simulink model "gm_soc_dvbs2_fpga"  (R2025b)
settings: Solver=VariableStepAuto  StartTime=0.0  StopTime=10.0  RelTol=1e-3
InitFcn:
  | soc_dvbs2_init;
undefined symbols (not defined in the file or in its folder): Add, coefficientsLog, coefficientsSqrt1, coefficientsSqrt2, dataBits, Deinterleaver, designMultirateFIR, noisePow, Shift, Short, soc_dvbs2_designFIRFilter, soc_dvbs2_txPacketBits, syncWord, txDataOut, txFiltCoeff, XData
libraries: simulink x304, hdlsllib x265, dspsigops x15, dsphdlfiltering2 x8, hdlmdlgenlib x6, dsphdlsigops2 x5, commseqgen3 x5, dsphdlmathfun2 x3, hwlogicconnlib x2, whdledac x2, commhdlcrc x2, whdlutilities x1
(part 16 of 36)

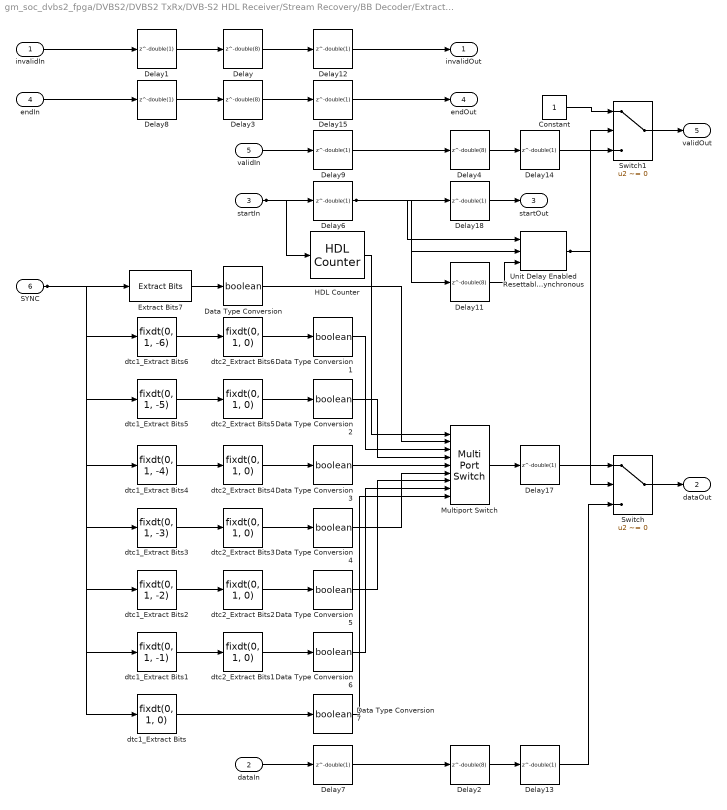
== system gm_soc_dvbs2_fpga/DVBS2/DVBS2 TxRx/DVB-S2 HDL Receiver/Stream Recovery/BB Decoder/Extract Stream/Insert SYNC ==
  invalidIn : Inport  OutDataTypeStr=boolean  PortDimensions=1  SampleTime=7.8125e-09
  dataIn : Inport  Port=2  OutDataTypeStr=boolean  PortDimensions=1  SampleTime=7.8125e-09
  startIn : Inport  Port=3  OutDataTypeStr=boolean  PortDimensions=1  SampleTime=7.8125e-09
  endIn : Inport  Port=4  OutDataTypeStr=boolean  PortDimensions=1  SampleTime=7.8125e-09
  validIn : Inport  Port=5  OutDataTypeStr=boolean  PortDimensions=1  SampleTime=7.8125e-09
  SYNC : Inport  Port=6  OutDataTypeStr=uint8  PortDimensions=1  SampleTime=7.8125e-09
  Constant : Constant  OutDataTypeStr=boolean  SampleTime=7.8125e-09
  Data Type Conversion{,1..7} (8 alike) : DataTypeConversion  OutDataTypeStr=boolean  SampleTime=7.8125e-09  SaturateOnIntegerOverflow=off  RndMeth=Floor
  Delay{,2..4,11} (5 alike) : Delay  DelayLength=double(8)  InitialCondition=0  SampleTime=7.8125e-09
  Delay{1,6..9,12..15,17..18} (11 alike) : Delay  DelayLength=double(1)  InitialCondition=0  SampleTime=7.8125e-09
  Extract Bits7 : simulink/Logic and Bit Operations/Extract Bits  bitsToExtract=Range of bits  numBits=8  bitIdxRange=[7 7]  outScalingMode=Treat bit field as an integer
  HDL Counter : hdlsllib/Sources/HDL Counter  CountType=Count limited  CountInit=0  CountStep=1  CountMax=7  CountFromType=Initial value  CountFrom=0  CountResetPort=on  CountLoadPort=off  CountEnbPort=off  CountDirPort=off  CountHitOutputPort=off  CountDataType=Unsigned  CountWordLen=3  CountFracLen=0  CountSampTime=1
  Multiport Switch : MultiPortSwitch  DataPortOrder=Zero-based contiguous  Inputs=8  DiagnosticForDefault=None  zeroidx=on  SampleTime=7.8125e-09  SaturateOnIntegerOverflow=off  InputSameDT=off
  Switch : Switch  Criteria=u2 ~= 0  Threshold="fi(0,0,1,0,\"hex\",\"0\")"  OutDataTypeStr=boolean  SampleTime=7.8125e-09  SaturateOnIntegerOverflow=off  InputSameDT=off
  Switch1 : Switch  Criteria=u2 ~= 0  Threshold="fi(0,0,1,0,\"hex\",\"0\")"  OutDataTypeStr=boolean  SampleTime=7.8125e-09  SaturateOnIntegerOverflow=off  InputSameDT=off
  Unit Delay Enabled Resettable Synchronous : hdlsllib/Discrete/Unit Delay Enabled Resettable Synchronous  InitialCondition=double(0)  SampleTime=-1
  dtc1_Extract Bits : DataTypeConversion  OutDataTypeStr=fixdt(0, 1, 0)  SampleTime=7.8125e-09  SaturateOnIntegerOverflow=off  RndMeth=Floor
  dtc1_Extract Bits1 : DataTypeConversion  OutDataTypeStr=fixdt(0, 1, -1)  SampleTime=7.8125e-09  SaturateOnIntegerOverflow=off  RndMeth=Floor
  dtc1_Extract Bits2 : DataTypeConversion  OutDataTypeStr=fixdt(0, 1, -2)  SampleTime=7.8125e-09  SaturateOnIntegerOverflow=off  RndMeth=Floor
  dtc1_Extract Bits3 : DataTypeConversion  OutDataTypeStr=fixdt(0, 1, -3)  SampleTime=7.8125e-09  SaturateOnIntegerOverflow=off  RndMeth=Floor
  dtc1_Extract Bits4 : DataTypeConversion  OutDataTypeStr=fixdt(0, 1, -4)  SampleTime=7.8125e-09  SaturateOnIntegerOverflow=off  RndMeth=Floor
  dtc1_Extract Bits5 : DataTypeConversion  OutDataTypeStr=fixdt(0, 1, -5)  SampleTime=7.8125e-09  SaturateOnIntegerOverflow=off  RndMeth=Floor
  dtc1_Extract Bits6 : DataTypeConversion  OutDataTypeStr=fixdt(0, 1, -6)  SampleTime=7.8125e-09  SaturateOnIntegerOverflow=off  RndMeth=Floor
  dtc2_Extract Bits{1..6} (6 alike) : DataTypeConversion  OutDataTypeStr=fixdt(0, 1, 0)  ConvertRealWorld=Stored Integer (SI)  SampleTime=7.8125e-09  SaturateOnIntegerOverflow=off  RndMeth=Floor
  invalidOut : Outport  SampleTime=7.8125e-09
  dataOut : Outport  Port=2  SampleTime=7.8125e-09
  startOut : Outport  Port=3  SampleTime=7.8125e-09
  endOut : Outport  Port=4  SampleTime=7.8125e-09
  validOut : Outport  Port=5  SampleTime=7.8125e-09
  wires:
  dtc1_Extract Bits5/1 -> dtc2_Extract Bits5/1
  Data Type Conversion3/1 -> Multiport Switch/5
  Delay/1 -> Delay12/1
  dtc1_Extract Bits6/1 -> dtc2_Extract Bits6/1
  Data Type Conversion7/1 -> Multiport Switch/9
  invalidIn/1 -> Delay1/1
  dtc2_Extract Bits2/1 -> Data Type Conversion5/1
  SYNC/1 -> dtc1_Extract Bits6/1, dtc1_Extract Bits4/1, Extract Bits7/1, dtc1_Extract Bits3/1, dtc1_Extract Bits2/1, dtc1_Extract Bits1/1, dtc1_Extract Bits5/1, dtc1_Extract Bits/1
  Data Type Conversion6/1 -> Multiport Switch/8
  endIn/1 -> Delay8/1
  Delay12/1 -> invalidOut/1
  Delay1/1 -> Delay/1
  Delay8/1 -> Delay3/1
  Extract Bits7/1 -> Data Type Conversion/1
  dtc1_Extract Bits4/1 -> dtc2_Extract Bits4/1
  dtc1_Extract Bits3/1 -> dtc2_Extract Bits3/1
  validIn/1 -> Delay9/1
  dtc1_Extract Bits2/1 -> dtc2_Extract Bits2/1
  dtc1_Extract Bits1/1 -> dtc2_Extract Bits1/1
  dtc1_Extract Bits/1 -> Data Type Conversion7/1
  Delay3/1 -> Delay15/1
  Data Type Conversion5/1 -> Multiport Switch/7
  startIn/1 -> Delay6/1, HDL Counter/1
  Data Type Conversion/1 -> Multiport Switch/2
  Data Type Conversion4/1 -> Multiport Switch/6
  dtc2_Extract Bits6/1 -> Data Type Conversion1/1
  Data Type Conversion2/1 -> Multiport Switch/4
  dtc2_Extract Bits5/1 -> Data Type Conversion2/1
  dataIn/1 -> Delay7/1
  dtc2_Extract Bits4/1 -> Data Type Conversion3/1
  Constant/1 -> Switch1/1
  dtc2_Extract Bits3/1 -> Data Type Conversion4/1
  dtc2_Extract Bits1/1 -> Data Type Conversion6/1
  Delay15/1 -> endOut/1
  Delay9/1 -> Delay4/1
  Delay6/1 -> Unit Delay Enabled Resettable Synchronous/1, Unit Delay Enabled Resettable Synchronous/2, Delay18/1, Delay11/1
  HDL Counter/1 -> Multiport Switch/1
  Data Type Conversion1/1 -> Multiport Switch/3
  Delay7/1 -> Delay2/1
  Unit Delay Enabled Resettable Synchronous/1 -> Switch1/2, Switch/2
  Delay4/1 -> Delay14/1
  Delay18/1 -> startOut/1
  Switch1/1 -> validOut/1
  Delay11/1 -> Unit Delay Enabled Resettable Synchronous/3
  Multiport Switch/1 -> Delay17/1
  Delay2/1 -> Delay13/1
  Delay14/1 -> Switch1/3
  Delay17/1 -> Switch/1
  Delay13/1 -> Switch/3
  Switch/1 -> dataOut/1

== system gm_soc_dvbs2_fpga/DVBS2/DVBS2 TxRx/DVB-S2 HDL Receiver/Synchronizer and PL Header Decoder/Fine Phase Synchronizer/Power Q and Beta Offset Rotation/Complex Multiplier ==
  In1 : Inport  OutDataTypeStr=fixdt(1, 22, 14)  PortDimensions=1  SampleTime=2.5e-07
      settings: SignalType=complex
  In2 : Inport  Port=2  OutDataTypeStr=fixdt(1, 22, 14)  PortDimensions=1  SampleTime=2.5e-07
      settings: SignalType=complex
  AddADn : Sum  Inputs=++|  OutDataTypeStr=fixdt(1, 22, 14)
  AddAUp : Sum  Inputs=|+-  OutDataTypeStr=fixdt(1, 22, 14)
  AddBCtr : Sum  Inputs=+|+  OutDataTypeStr=fixdt(1, 23, 14)
  AddBDn : Sum  Inputs=|+-  OutDataTypeStr=fixdt(1, 23, 14)
  AddBUp : Sum  Inputs=++|  OutDataTypeStr=fixdt(1, 23, 14)
  Complex to Real-Imag : ComplexToRealImag
  Complex to Real-Imag1 : ComplexToRealImag
  Delay{1..8,21} (9 alike) : Delay
  Delay{9..20} (12 alike) : Delay  DelayLength=1
  ProductCtr : Product  OutDataTypeStr=fixdt(1, 45, 28)
  ProductDn : Product  OutDataTypeStr=fixdt(1, 45, 28)
  ProductUp : Product  OutDataTypeStr=fixdt(1, 45, 28)
  Real-Imag to Complex : RealImagToComplex
  Out1 : Outport  SampleTime=2.5e-07  VectorParamsAs1DForOutWhenUnconnected=off
  wires:
  Delay9/1 -> AddBUp/1
  Delay7/1 -> Delay17/1
  ProductUp/1 -> Delay21/1
  AddBDn/1 -> Delay5/1
  [IM2] -> Delay15/1
  [RE2] -> Delay14/1
  Delay5/1 -> ProductDn/2
  [IM2] -> Delay10/1
  AddAUp/1 -> Delay19/1
  ProductCtr/1 -> Delay7/1
  Complex to Real-Imag/2 -> Delay13/1
  [RE2] -> Delay9/1
  Delay11/1 -> AddBCtr/1, Delay1/1
  In1/1 -> Complex to Real-Imag/1
  Delay10/1 -> AddBUp/2
  Delay12/1 -> Delay3/1
  In2/1 -> Complex to Real-Imag1/1
  Complex to Real-Imag/1 -> Delay11/1
  Complex to Real-Imag1/1 -> [RE2]
  Complex to Real-Imag1/2 -> [IM2]
  Delay14/1 -> AddBDn/1
  Delay15/1 -> AddBDn/2
  AddADn/1 -> Delay20/1
  AddBUp/1 -> Delay8/1
  ProductDn/1 -> Delay6/1
  AddBCtr/1 -> Delay2/1
  [IM2] -> Delay12/1
  Delay13/1 -> AddBCtr/2, Delay4/1
  Delay8/1 -> ProductUp/1
  Delay1/1 -> ProductUp/2
  Delay4/1 -> ProductDn/1
  Delay2/1 -> ProductCtr/1
  Delay3/1 -> ProductCtr/2
  Delay21/1 -> Delay16/1
  Delay6/1 -> Delay18/1
  Delay18/1 -> AddADn/2
  Delay16/1 -> AddAUp/1
  Delay17/1 -> AddAUp/2, AddADn/1
  Delay19/1 -> Real-Imag to Complex/1
  Delay20/1 -> Real-Imag to Complex/2
  Real-Imag to Complex/1 -> Out1/1

== system gm_soc_dvbs2_fpga/DVBS2/DVBS2 TxRx/DVB-S2 HDL Receiver/Synchronizer and PL Header Decoder/Fine Phase Synchronizer/Power Q and Beta Offset Rotation/Complex Multiplier1 ==
  In1 : Inport  OutDataTypeStr=fixdt(1, 22, 14)  PortDimensions=1  SampleTime=2.5e-07
      settings: SignalType=complex
  In2 : Inport  Port=2  OutDataTypeStr=fixdt(1, 22, 14)  PortDimensions=1  SampleTime=2.5e-07
      settings: SignalType=complex
  AddADn : Sum  Inputs=++|  OutDataTypeStr=fixdt(1, 22, 14)
  AddAUp : Sum  Inputs=|+-  OutDataTypeStr=fixdt(1, 22, 14)
  AddBCtr : Sum  Inputs=+|+  OutDataTypeStr=fixdt(1, 23, 14)
  AddBDn : Sum  Inputs=|+-  OutDataTypeStr=fixdt(1, 23, 14)
  AddBUp : Sum  Inputs=++|  OutDataTypeStr=fixdt(1, 23, 14)
  Complex to Real-Imag : ComplexToRealImag
  Complex to Real-Imag1 : ComplexToRealImag
  Delay{1..8,21} (9 alike) : Delay
  Delay{9..20} (12 alike) : Delay  DelayLength=1
  ProductCtr : Product  OutDataTypeStr=fixdt(1, 45, 28)
  ProductDn : Product  OutDataTypeStr=fixdt(1, 45, 28)
  ProductUp : Product  OutDataTypeStr=fixdt(1, 45, 28)
  Real-Imag to Complex : RealImagToComplex
  Out1 : Outport  SampleTime=2.5e-07  VectorParamsAs1DForOutWhenUnconnected=off
  wires:
  Real-Imag to Complex/1 -> Out1/1
  ProductUp/1 -> Delay21/1
  AddBDn/1 -> Delay5/1
  [IM2] -> Delay15/1
  [RE2] -> Delay14/1
  [IM2] -> Delay10/1
  AddAUp/1 -> Delay19/1
  ProductCtr/1 -> Delay7/1
  Complex to Real-Imag/2 -> Delay13/1
  [RE2] -> Delay9/1
  In1/1 -> Complex to Real-Imag/1
  Delay10/1 -> AddBUp/2
  Delay12/1 -> Delay3/1
  In2/1 -> Complex to Real-Imag1/1
  Delay20/1 -> Real-Imag to Complex/2
  Delay9/1 -> AddBUp/1
  Complex to Real-Imag/1 -> Delay11/1
  Complex to Real-Imag1/1 -> [RE2]
  ProductDn/1 -> Delay6/1
  AddBCtr/1 -> Delay2/1
  [IM2] -> Delay12/1
  Complex to Real-Imag1/2 -> [IM2]
  Delay14/1 -> AddBDn/1
  Delay15/1 -> AddBDn/2
  AddADn/1 -> Delay20/1
  AddBUp/1 -> Delay8/1
  Delay19/1 -> Real-Imag to Complex/1
  Delay11/1 -> AddBCtr/1, Delay1/1
  Delay13/1 -> AddBCtr/2, Delay4/1
  Delay8/1 -> ProductUp/1
  Delay1/1 -> ProductUp/2
  Delay4/1 -> ProductDn/1
  Delay5/1 -> ProductDn/2
  Delay2/1 -> ProductCtr/1
  Delay3/1 -> ProductCtr/2
  Delay21/1 -> Delay16/1
  Delay6/1 -> Delay18/1
  Delay16/1 -> AddAUp/1
  Delay7/1 -> Delay17/1
  Delay17/1 -> AddAUp/2, AddADn/1
  Delay18/1 -> AddADn/2

== system gm_soc_dvbs2_fpga/DVBS2/DVBS2 TxRx/DVB-S2 HDL Receiver/Synchronizer and PL Header Decoder/Fine Phase Synchronizer/Power Q and Beta Offset Rotation/Complex Multiplier2 ==
  In1 : Inport  OutDataTypeStr=fixdt(1, 22, 14)  PortDimensions=1  SampleTime=2.5e-07
      settings: SignalType=complex
  In2 : Inport  Port=2  OutDataTypeStr=fixdt(1, 22, 14)  PortDimensions=1  SampleTime=2.5e-07
      settings: SignalType=complex
  AddADn : Sum  Inputs=++|  OutDataTypeStr=fixdt(1, 22, 14)
  AddAUp : Sum  Inputs=|+-  OutDataTypeStr=fixdt(1, 22, 14)
  AddBCtr : Sum  Inputs=+|+  OutDataTypeStr=fixdt(1, 23, 14)
  AddBDn : Sum  Inputs=|+-  OutDataTypeStr=fixdt(1, 23, 14)
  AddBUp : Sum  Inputs=++|  OutDataTypeStr=fixdt(1, 23, 14)
  Complex to Real-Imag : ComplexToRealImag
  Complex to Real-Imag1 : ComplexToRealImag
  Delay{1..8,21} (9 alike) : Delay
  Delay{9..20} (12 alike) : Delay  DelayLength=1
  ProductCtr : Product  OutDataTypeStr=fixdt(1, 45, 28)
  ProductDn : Product  OutDataTypeStr=fixdt(1, 45, 28)
  ProductUp : Product  OutDataTypeStr=fixdt(1, 45, 28)
  Real-Imag to Complex : RealImagToComplex
  Out1 : Outport  SampleTime=2.5e-07  VectorParamsAs1DForOutWhenUnconnected=off
  wires:
  Delay20/1 -> Real-Imag to Complex/2
  Delay9/1 -> AddBUp/1
  Delay7/1 -> Delay17/1
  [IM2] -> Delay15/1
  [RE2] -> Delay14/1
  Delay5/1 -> ProductDn/2
  [IM2] -> Delay10/1
  [RE2] -> Delay9/1
  In1/1 -> Complex to Real-Imag/1
  In2/1 -> Complex to Real-Imag1/1
  Delay10/1 -> AddBUp/2
  Complex to Real-Imag/1 -> Delay11/1
  AddAUp/1 -> Delay19/1
  ProductCtr/1 -> Delay7/1
  Complex to Real-Imag/2 -> Delay13/1
  Complex to Real-Imag1/1 -> [RE2]
  ProductDn/1 -> Delay6/1
  AddBCtr/1 -> Delay2/1
  Complex to Real-Imag1/2 -> [IM2]
  Delay14/1 -> AddBDn/1
  Delay15/1 -> AddBDn/2
  AddADn/1 -> Delay20/1
  AddBUp/1 -> Delay8/1
  Delay19/1 -> Real-Imag to Complex/1
  Delay11/1 -> AddBCtr/1, Delay1/1
  [IM2] -> Delay12/1
  Delay13/1 -> AddBCtr/2, Delay4/1
  Real-Imag to Complex/1 -> Out1/1
  ProductUp/1 -> Delay21/1
  AddBDn/1 -> Delay5/1
  Delay8/1 -> ProductUp/1
  Delay1/1 -> ProductUp/2
  Delay12/1 -> Delay3/1
  Delay4/1 -> ProductDn/1
  Delay2/1 -> ProductCtr/1
  Delay3/1 -> ProductCtr/2
  Delay21/1 -> Delay16/1
  Delay6/1 -> Delay18/1
  Delay18/1 -> AddADn/2
  Delay16/1 -> AddAUp/1
  Delay17/1 -> AddAUp/2, AddADn/1

== system gm_soc_dvbs2_fpga/DVBS2/DVBS2 TxRx/DVB-S2 HDL Receiver/Synchronizer and PL Header Decoder/Fine Phase Synchronizer/Power Q and Beta Offset Rotation/Gain ==
  In1 : Inport  OutDataTypeStr=fixdt(1, 22, 14)  PortDimensions=1  SampleTime=2.5e-07
      settings: SignalType=complex
  AddADn : Sum  Inputs=++|  OutDataTypeStr=fixdt(1, 22, 14)
  AddAUp : Sum  Inputs=|+-  OutDataTypeStr=fixdt(1, 22, 14)
  AddBCtr : Sum  Inputs=+|+  OutDataTypeStr=fixdt(1, 23, 14)
  AddBDn : Sum  Inputs=|+-  OutDataTypeStr=fixdt(1, 17, 15)
  AddBUp : Sum  Inputs=++|  OutDataTypeStr=fixdt(1, 17, 15)
  Complex to Real-Imag : ComplexToRealImag
  Complex to Real-Imag1 : ComplexToRealImag
  Constant : Constant  Value=fi(exp(1i*pi/4),1,16)  OutDataTypeStr=fixdt(1, 16, 15)  SampleTime=-1
  Delay{1..8,21} (9 alike) : Delay
  Delay{9..20} (12 alike) : Delay  DelayLength=1
  ProductCtr : Product  OutDataTypeStr=fixdt(1, 39, 29)
  ProductDn : Product  OutDataTypeStr=fixdt(1, 39, 29)
  ProductUp : Product  OutDataTypeStr=fixdt(1, 39, 29)
  Real-Imag to Complex : RealImagToComplex
  Out1 : Outport  SampleTime=2.5e-07  VectorParamsAs1DForOutWhenUnconnected=off
  wires:
  Delay9/1 -> AddBUp/1
  Delay7/1 -> Delay17/1
  ProductUp/1 -> Delay21/1
  [IM2] -> Delay15/1
  Delay20/1 -> Real-Imag to Complex/2
  [RE2] -> Delay14/1
  Delay5/1 -> ProductDn/2
  [IM2] -> Delay10/1
  ProductCtr/1 -> Delay7/1
  [RE2] -> Delay9/1
  Delay10/1 -> AddBUp/2
  Constant/1 -> Complex to Real-Imag1/1
  In1/1 -> Complex to Real-Imag/1
  Complex to Real-Imag/1 -> Delay11/1
  AddAUp/1 -> Delay19/1
  Complex to Real-Imag/2 -> Delay13/1
  Complex to Real-Imag1/1 -> [RE2]
  AddBCtr/1 -> Delay2/1
  Complex to Real-Imag1/2 -> [IM2]
  Delay14/1 -> AddBDn/1
  Delay15/1 -> AddBDn/2
  AddBUp/1 -> Delay8/1
  Delay11/1 -> Delay1/1, AddBCtr/1
  ProductDn/1 -> Delay6/1
  [IM2] -> Delay12/1
  Delay13/1 -> AddBCtr/2, Delay4/1
  Real-Imag to Complex/1 -> Out1/1
  AddBDn/1 -> Delay5/1
  Delay8/1 -> ProductUp/1
  Delay1/1 -> ProductUp/2
  Delay12/1 -> Delay3/1
  Delay4/1 -> ProductDn/1
  Delay2/1 -> ProductCtr/1
  AddADn/1 -> Delay20/1
  Delay3/1 -> ProductCtr/2
  Delay21/1 -> Delay16/1
  Delay6/1 -> Delay18/1
  Delay16/1 -> AddAUp/1
  Delay17/1 -> AddADn/1, AddAUp/2
  Delay18/1 -> AddADn/2
  Delay19/1 -> Real-Imag to Complex/1

== system gm_soc_dvbs2_fpga/DVBS2/DVBS2 TxRx/DVB-S2 HDL Receiver/Synchronizer and PL Header Decoder/Fine Phase Synchronizer/Power Q and Beta Offset Rotation/Gain1 ==
  In1 : Inport  OutDataTypeStr=fixdt(1, 22, 14)  PortDimensions=1  SampleTime=2.5e-07
      settings: SignalType=complex
  AddADn : Sum  Inputs=++|  OutDataTypeStr=fixdt(1, 22, 14)
  AddAUp : Sum  Inputs=|+-  OutDataTypeStr=fixdt(1, 22, 14)
  AddBCtr : Sum  Inputs=+|+  OutDataTypeStr=fixdt(1, 23, 14)
  AddBDn : Sum  Inputs=|+-  OutDataTypeStr=fixdt(1, 17, 15)
  AddBUp : Sum  Inputs=++|  OutDataTypeStr=fixdt(1, 17, 15)
  Complex to Real-Imag : ComplexToRealImag
  Complex to Real-Imag1 : ComplexToRealImag
  Constant : Constant  Value=fi(exp(1i*pi/4),1,16)  OutDataTypeStr=fixdt(1, 16, 15)  SampleTime=-1
  Delay{1..8,21} (9 alike) : Delay
  Delay{9..20} (12 alike) : Delay  DelayLength=1
  ProductCtr : Product  OutDataTypeStr=fixdt(1, 39, 29)
  ProductDn : Product  OutDataTypeStr=fixdt(1, 39, 29)
  ProductUp : Product  OutDataTypeStr=fixdt(1, 39, 29)
  Real-Imag to Complex : RealImagToComplex
  Out1 : Outport  SampleTime=2.5e-07  VectorParamsAs1DForOutWhenUnconnected=off
  wires:
  Delay9/1 -> AddBUp/1
  Delay7/1 -> Delay17/1
  ProductUp/1 -> Delay21/1
  AddBDn/1 -> Delay5/1
  [IM2] -> Delay15/1
  [RE2] -> Delay14/1
  Delay5/1 -> ProductDn/2
  [IM2] -> Delay10/1
  AddAUp/1 -> Delay19/1
  ProductCtr/1 -> Delay7/1
  [RE2] -> Delay9/1
  Delay10/1 -> AddBUp/2
  Constant/1 -> Complex to Real-Imag1/1
  In1/1 -> Complex to Real-Imag/1
  Complex to Real-Imag/1 -> Delay11/1
  Complex to Real-Imag/2 -> Delay13/1
  Complex to Real-Imag1/1 -> [RE2]
  Complex to Real-Imag1/2 -> [IM2]
  Delay14/1 -> AddBDn/1
  Delay15/1 -> AddBDn/2
  AddBUp/1 -> Delay8/1
  Delay11/1 -> AddBCtr/1, Delay1/1
  ProductDn/1 -> Delay6/1
  AddBCtr/1 -> Delay2/1
  [IM2] -> Delay12/1
  Delay13/1 -> AddBCtr/2, Delay4/1
  Delay8/1 -> ProductUp/1
  Delay1/1 -> ProductUp/2
  Delay12/1 -> Delay3/1
  Delay4/1 -> ProductDn/1
  Delay2/1 -> ProductCtr/1
  AddADn/1 -> Delay20/1
  Delay3/1 -> ProductCtr/2
  Delay19/1 -> Real-Imag to Complex/1
  Delay21/1 -> Delay16/1
  Delay6/1 -> Delay18/1
  Delay16/1 -> AddAUp/1
  Delay17/1 -> AddADn/1, AddAUp/2
  Delay20/1 -> Real-Imag to Complex/2
  Delay18/1 -> AddADn/2
  Real-Imag to Complex/1 -> Out1/1

== system gm_soc_dvbs2_fpga/DVBS2/DVBS2 TxRx/DVB-S2 HDL Receiver/Synchronizer and PL Header Decoder/PL Header Recovery/PL Header Decoder/Bit Flipping and Averaging ==
  dataIn : Inport  OutDataTypeStr=fixdt(1, 18, 13)  PortDimensions=1  SampleTime=2.5e-07
  indexIndicater : Inport  Port=2  OutDataTypeStr=boolean  PortDimensions=1  SampleTime=2.5e-07
  validIn : Inport  Port=3  OutDataTypeStr=boolean  PortDimensions=1  SampleTime=2.5e-07
  resetIn : Inport  Port=4  OutDataTypeStr=boolean  PortDimensions=1  SampleTime=2.5e-07
  hasPilots : Inport  Port=5  OutDataTypeStr=boolean  PortDimensions=1  SampleTime=2.5e-07
  Add : Sum  OutDataTypeStr=fixdt(1, 18, 13)
  Delay{1..14} (14 alike) : Delay
  Delay{15..23} (9 alike) : Delay  DelayLength=1
  Gain : Gain  Gain=1/2  ParamDataTypeStr=fixdt(0,1,1)  OutDataTypeStr=fixdt(1, 18, 13)
  Gain1 : Gain  Gain=-1  ParamDataTypeStr=fixdt(1,2,0)  OutDataTypeStr=fixdt(1, 18, 13)
  Logical Operator : Logic  AllPortsSameDT=off  OutDataTypeStr=boolean
  Logical Operator1 : Logic  AllPortsSameDT=off  OutDataTypeStr=boolean
  Logical Operator2 : Logic  Operator=NOT  AllPortsSameDT=off  OutDataTypeStr=boolean
  Switch1 : Switch  Criteria=u2 ~= 0  OutDataTypeStr=fixdt(1, 18, 13)  SaturateOnIntegerOverflow=off  InputSameDT=off
  Switch2 : Switch  Criteria=u2 ~= 0  OutDataTypeStr=fixdt(1, 18, 13)  SaturateOnIntegerOverflow=off  InputSameDT=off
  Unit Delay Enabled Synchronous : hdlsllib/Discrete/Unit Delay Enabled Synchronous  InitialCondition=0.0  SampleTime=-1
  dataOut : Outport  SampleTime=2.5e-07
  validOut : Outport  Port=2  SampleTime=2.5e-07
  resetOut : Outport  Port=3  SampleTime=2.5e-07
  wires:
  validIn/1 -> Delay10/1
  dataIn/1 -> Delay4/1, Delay3/1
  Delay11/1 -> Delay14/1
  Delay1/1 -> Switch1/1
  resetIn/1 -> Delay11/1
  Gain1/1 -> Delay1/1
  Delay3/1 -> Gain1/1
  indexIndicater/1 -> Delay9/1, Delay6/1
  Delay4/1 -> Delay2/1
  Delay6/1 -> Delay5/1
  Delay10/1 -> Delay13/1
  hasPilots/1 -> Delay7/1
  Delay9/1 -> Delay12/1
  Delay14/1 -> Delay20/1
  Delay5/1 -> Switch1/2
  Delay2/1 -> Delay17/1, Switch1/3
  Delay7/1 -> Delay8/1
  Delay12/1 -> Delay18/1
  Delay13/1 -> Delay19/1
  Delay20/1 -> Delay23/1
  Switch1/1 -> Delay15/1
  Logical Operator/1 -> Delay22/1
  Delay8/1 -> Delay16/1
  Delay18/1 -> Logical Operator2/1, Logical Operator/1
  Delay19/1 -> Logical Operator1/2, Logical Operator/2
  Delay23/1 -> resetOut/1
  Delay15/1 -> Switch2/1
  Delay16/1 -> Switch2/2
  Delay17/1 -> Switch2/3
  Logical Operator2/1 -> Logical Operator1/1
  Switch2/1 -> Gain/1
  Logical Operator1/1 -> Unit Delay Enabled Synchronous/2
  Delay22/1 -> validOut/1
  Gain/1 -> Add/1, Unit Delay Enabled Synchronous/1
  Unit Delay Enabled Synchronous/1 -> Add/2
  Add/1 -> Delay21/1
  Delay21/1 -> dataOut/1
